simulink model "perturb_lateral"  (R2022b)
settings: Solver=VariableStepAuto  StartTime=0.0  StopTime=10.0  RelTol=1e-3
undefined symbols (not defined in the file or in its folder): m
settings Model: Creator=aceao  LastModifiedBy=aceao

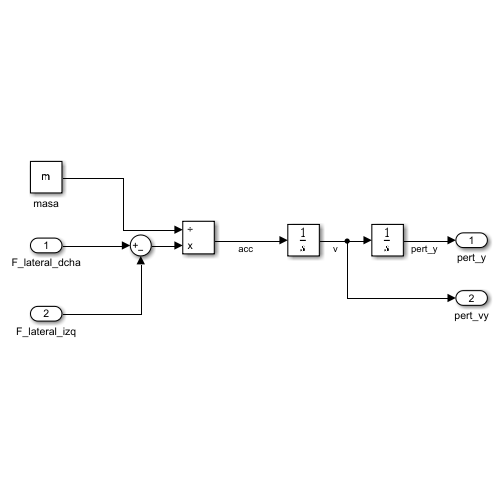
[thumbnail: Simulink's stored preview of the top-level diagram]
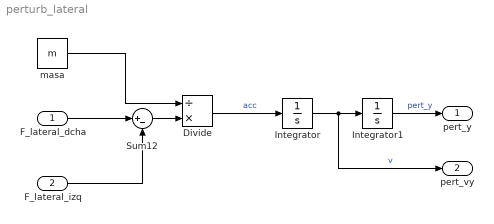
== system perturb_lateral ==
  F_lateral_dcha : Inport
  F_lateral_izq : Inport  Port=2
  Divide : Product  Inputs=/*
  Integrator : Integrator
  Integrator1 : Integrator
  Sum12 : Sum  Inputs=|+-
  masa : Constant  Value=m
  pert_y : Outport
  pert_vy : Outport  Port=2
  wires:
  Integrator/1 -> pert_vy/1, Integrator1/1  "v"
  F_lateral_izq/1 -> Sum12/2
  F_lateral_dcha/1 -> Sum12/1
  Sum12/1 -> Divide/2
  Divide/1 -> Integrator/1  "acc"
  masa/1 -> Divide/1
  Integrator1/1 -> pert_y/1  "pert_y"
